simulink model "sampleModel92"  (R2021b)
settings: Solver=VariableStepAuto  StartTime=0.0  StopTime=10.0  RelTol=1e-3
undefined symbols (not defined in the file or in its folder): DiscIntNeverNeededParam, Newton, Raphson
libraries: simulink x6
settings Model: Creator=user  LastModifiedBy=user

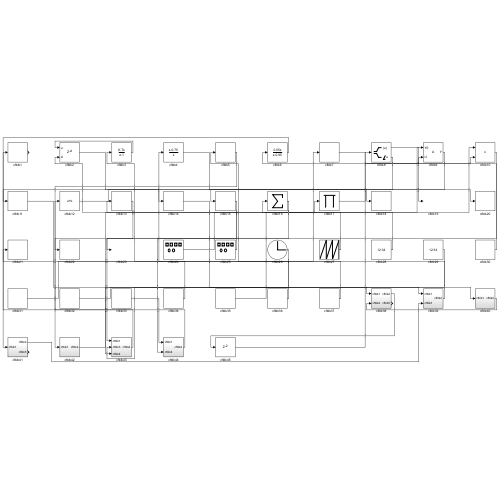
[thumbnail: Simulink's stored preview of the top-level diagram]
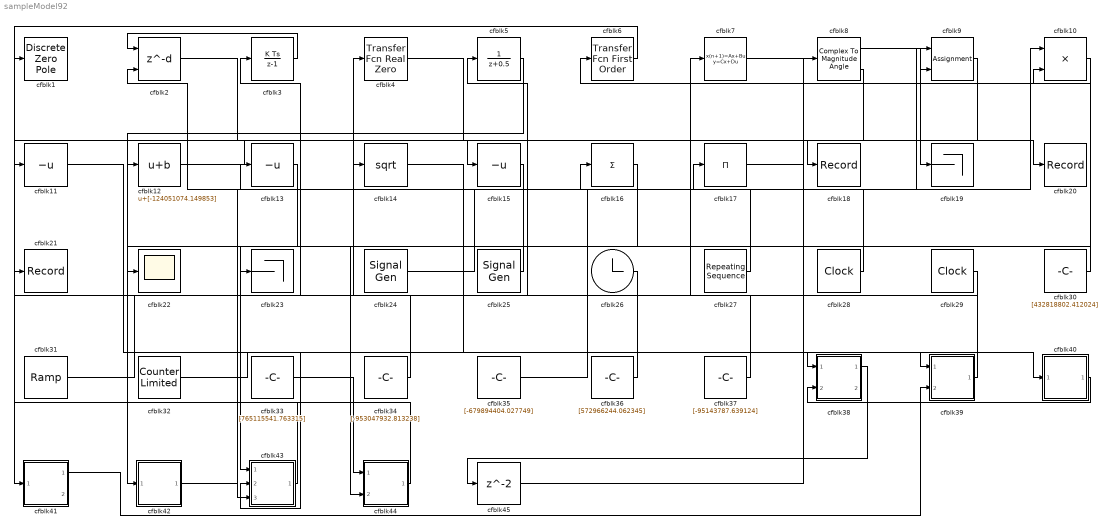
== system sampleModel92 ==
  cfblk1 : DiscreteZeroPole  Poles=[0 0.5]  Gain=1
  cfblk10 : Product
  cfblk11 : UnaryMinus
  cfblk12 : Bias  Bias=[-124051074.149853]
  cfblk13 : UnaryMinus
  cfblk14 : Sqrt  SaturateOnIntegerOverflow=on
  cfblk15 : UnaryMinus
  cfblk16 : Sum  Inputs=+
  cfblk17 : Product  Inputs=*
  cfblk18 : Record  FileSettingsInternal="{\"entries\":[{\"content\":{\"excelSettings\":{\"content\":{},\"type\":\"Streamout.ExcelSettings\"}},\"type\":\"Streamout.FileSettingStorage\",\"uuid\":\"6a51076d-8da9-4467-914a-28448b775d9d\"}],\"packageUris\":[\"http://schema.mathworks.com/mf0/streamout_blocks/R2020a\"],\"version\":\"1.0\"}"  SignalsInternal="{\"entries\":[{\"content\":{\"signals\":[{\"content\":{\"blockPath\":[\"sampleModel92/cfblk18\"],\"channel\":[],\"dimensions\":[1],\"domain\":\"sampleModel92/cfblk18\",\"lineColor\":\"#7e2f8e\",\"plots\":[1],\"port\":1,\"sid\":[\"\"],\"signalID\":3336,\"signalName\":\"cfblk4\"},\"type\":\"RecordBlkView.Signal\",\"uuid\":\"c4f05d71-166b-4c34-8946-7f08c4cc9336\"}]},\"type\":\"RecordBlkView.InputSignals\",\"uuid\":\"7a531b9c-db59-4839-bb56-90dd1c5d6161\"}],\"packageUris\":[\"http://schema.mathworks.com/mf0/streamout_blocks/R2020a\"],\"version\":\"1.0\"}"  VisualizationBindings="{\"sparklinesplugin\":{\"info\":[{\"bindingParametersList\":[],\"subplotID\":1}]}}"
  cfblk19 : Terminator
  cfblk2 : Delay  DelayLengthSource=Input port  SampleTime=1
      settings: InputPortMap=u0,p1
  cfblk20 : Record  FileSettingsInternal="{\"entries\":[{\"content\":{\"excelSettings\":{\"content\":{},\"type\":\"Streamout.ExcelSettings\"}},\"type\":\"Streamout.FileSettingStorage\",\"uuid\":\"9044f618-eb01-48c3-80c5-be2844ab762f\"}],\"packageUris\":[\"http://schema.mathworks.com/mf0/streamout_blocks/R2020a\"],\"version\":\"1.0\"}"  SignalsInternal="{\"entries\":[{\"content\":{\"signals\":[{\"content\":{\"blockPath\":[\"sampleModel92/cfblk20\"],\"channel\":[],\"dimensions\":[1],\"domain\":\"sampleModel92/cfblk20\",\"lineColor\":\"#d95319\",\"plots\":[1],\"port\":1,\"sid\":[\"\"],\"signalID\":3328,\"signalName\":\"cfblk12\"},\"type\":\"RecordBlkView.Signal\",\"uuid\":\"913b886d-d33f-4f21-af18-8c6dc12f15ac\"}]},\"type\":\"RecordBlkView.InputSignals\",\"uuid\":\"b0a329a0-5a63-4f71-bd89-f24f022d2b5e\"}],\"packageUris\":[\"http://schema.mathworks.com/mf0/streamout_blocks/R2020a\"],\"version\":\"1.0\"}"  VisualizationBindings="{\"sparklinesplugin\":{\"info\":[{\"bindingParametersList\":[],\"subplotID\":1}]}}"
  cfblk21 : Record  FileSettingsInternal="{\"entries\":[{\"content\":{\"excelSettings\":{\"content\":{},\"type\":\"Streamout.ExcelSettings\"}},\"type\":\"Streamout.FileSettingStorage\",\"uuid\":\"8f3cd402-b646-49ca-a95d-ee623ab04474\"}],\"packageUris\":[\"http://schema.mathworks.com/mf0/streamout_blocks/R2020a\"],\"version\":\"1.0\"}"  SignalsInternal="{\"entries\":[{\"content\":{\"signals\":[{\"content\":{\"blockPath\":[\"sampleModel92/cfblk21\"],\"channel\":[],\"dimensions\":[1],\"domain\":\"sampleModel92/cfblk21\",\"lineColor\":\"#edb120\",\"plots\":[1],\"port\":1,\"sid\":[\"\"],\"signalID\":3332,\"signalName\":\"cfblk44\"},\"type\":\"RecordBlkView.Signal\",\"uuid\":\"ded4a17a-d02b-4987-8ca6-efb213871c75\"}]},\"type\":\"RecordBlkView.InputSignals\",\"uuid\":\"37dec361-af1f-4bc5-9898-b83d7289465a\"}],\"packageUris\":[\"http://schema.mathworks.com/mf0/streamout_blocks/R2020a\"],\"version\":\"1.0\"}"  VisualizationBindings="{\"sparklinesplugin\":{\"info\":[{\"bindingParametersList\":[],\"subplotID\":1}]}}"
  cfblk22 : Scope
  cfblk23 : Terminator
  cfblk24 : SignalGenerator  WaveForm=square  Amplitude=[-232298427.967946]  Units=rad/sec
  cfblk25 : SignalGenerator  Amplitude=[-137299027.507502]  Units=rad/sec
  cfblk26 : Clock
  cfblk27 : simulink/Sources/Repeating Sequence  rep_seq_t=[0 2]  rep_seq_y=[-945702141.819262, 64967850.415956]
  cfblk28 : DigitalClock
  cfblk29 : DigitalClock
  cfblk3 : DiscreteIntegrator  ICPrevOutput=DiscIntNeverNeededParam  ICPrevScaledInput=DiscIntNeverNeededParam
  cfblk30 : Constant  Value=[432818802.412024]  SampleTime=1
  cfblk31 : simulink/Sources/Ramp  slope=[-2473.565325]  start=[11.966407]  InitialOutput=[854978.820776]
  cfblk32 : simulink/Sources/Counter Limited  uplimit=[365.000000]  tsamp=-1
  cfblk33 : Constant  Value=[765115541.763315]  SampleTime=1
  cfblk34 : Constant  Value=[-953047932.813238]  SampleTime=1
  cfblk35 : Constant  Value=[-679894404.027749]  SampleTime=1
  cfblk36 : Constant  Value=[572966244.062345]  SampleTime=1
  cfblk37 : Constant  Value=[-95143787.639124]  SampleTime=1
  cfblk38 : Subsystem
  cfblk39 : Subsystem
  cfblk4 : simulink/Discrete/Transfer Fcn Real Zero  ZeroZ=0.75  ICPrevInput=0.0  DoSatur=off
      settings: SourceProductBaseCode=SL
  cfblk40 : Subsystem
  cfblk41 : Subsystem
  cfblk42 : Subsystem
  cfblk43 : Subsystem
  cfblk44 : Subsystem
  cfblk45 : Delay  SampleTime=1
  cfblk5 : DiscreteTransferFcn  SampleTime=1
  cfblk6 : simulink/Discrete/Transfer Fcn First Order  PoleZ=0.95  ICPrevOutput=0.0  DoSatur=off
  cfblk7 : DiscreteStateSpace
  cfblk8 : ComplexToMagnitudeAngle
  cfblk9 : Assignment  DiagnosticForDimensions=Warning  IndexOptions=Index vector (dialog)  Indices=1  OutputSizes=1
  wires:
  cfblk12/1 -> cfblk20/1
  cfblk15/1 -> cfblk43/1(cfblk1)
  cfblk30/1 -> cfblk6/1
  cfblk9/1 -> cfblk15/1
  cfblk26/1 -> cfblk43/2(cfblk3)
  cfblk5/1 -> cfblk42/1(cfblk1)
  cfblk24/1 -> cfblk10/1
  cfblk43/1(cfblk2) -> cfblk12/1
  cfblk36/1 -> cfblk5/1
  cfblk29/1 -> cfblk43/3(cfblk4)
  cfblk3/1 -> cfblk2/1
  cfblk8/1 -> cfblk19/1
  cfblk13/1 -> cfblk23/1
  cfblk25/1 -> cfblk13/1
  cfblk35/1 -> cfblk9/1
  cfblk4/1 -> cfblk18/1
  cfblk27/1 -> cfblk2/2
  cfblk6/1 -> cfblk41/1(cfblk1)
  cfblk37/1 -> cfblk1/1
  cfblk10/1 -> cfblk22/1
  cfblk32/1 -> cfblk40/1(cfblk1)
  cfblk28/1 -> cfblk16/1
  cfblk39/1(cfblk2) -> cfblk4/1
  cfblk14/1 -> cfblk39/1(cfblk1)
  cfblk41/1(cfblk2) -> cfblk39/2(cfblk3)
  cfblk34/1 -> cfblk3/1
  cfblk42/1(cfblk2) -> cfblk17/1
  cfblk11/1 -> cfblk38/1(cfblk1)
  cfblk40/1(cfblk2) -> cfblk38/2(cfblk4)
  cfblk31/1 -> cfblk7/1
  cfblk17/1 -> cfblk10/2
  cfblk2/1 -> cfblk14/1
  cfblk33/1 -> cfblk44/1(cfblk1)
  cfblk44/1(cfblk2) -> cfblk21/1
  cfblk7/1 -> cfblk9/2
  cfblk16/1 -> cfblk44/2(cfblk4)
  cfblk8/2 -> cfblk11/1
  cfblk38/1(cfblk2) -> cfblk45/1
  cfblk45/1 -> cfblk8/1

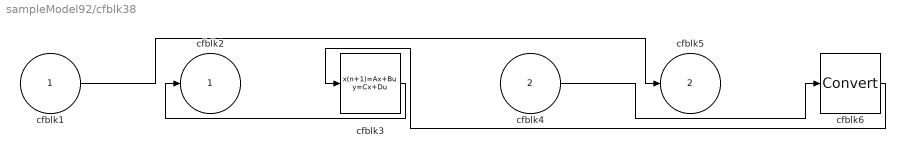
== system sampleModel92/cfblk38 ==
  cfblk1 : Inport
  cfblk4 : Inport  Port=2
  cfblk3 : DiscreteStateSpace
  cfblk6 : DataTypeConversion
  cfblk2 : Outport
  cfblk5 : Outport  Port=2
  wires:
  cfblk3/1 -> cfblk2/1
  cfblk1/1 -> cfblk5/1
  cfblk4/1 -> cfblk6/1
  cfblk6/1 -> cfblk3/1

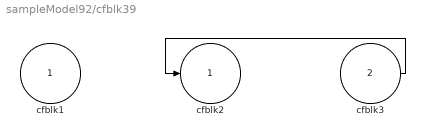
== system sampleModel92/cfblk39 ==
  cfblk1 : Inport
  cfblk3 : Inport  Port=2
  cfblk2 : Outport
  wires:
  cfblk3/1 -> cfblk2/1

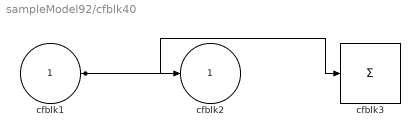
== system sampleModel92/cfblk40 ==
  cfblk1 : Inport
  cfblk3 : Sum  Inputs=+
  cfblk2 : Outport
  wires:
  cfblk1/1 -> cfblk2/1, cfblk3/1

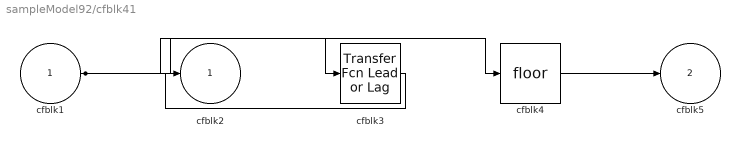
== system sampleModel92/cfblk41 ==
  cfblk1 : Inport
  cfblk3 : simulink/Discrete/Transfer Fcn Lead or Lag  PoleZ=0.95  ZeroZ=0.75  ICPrevOutput=0.0  ICPrevInput=0.0  DoSatur=off
      settings: SourceProductBaseCode=SL
  cfblk4 : Rounding
  cfblk2 : Outport
  cfblk5 : Outport  Port=2
  wires:
  cfblk1/1 -> cfblk4/1, cfblk3/1
  cfblk4/1 -> cfblk5/1
  cfblk3/1 -> cfblk2/1

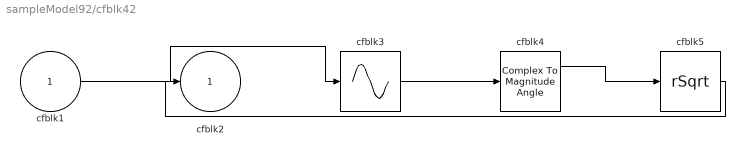
== system sampleModel92/cfblk42 ==
  cfblk1 : Inport
  cfblk3 : Sin  TimeSource=Use external signal  SampleTime=0
  cfblk4 : ComplexToMagnitudeAngle
  cfblk5 : Sqrt  Operator=rSqrt  AlgorithmType=Newton-Raphson  SaturateOnIntegerOverflow=on
  cfblk2 : Outport
  wires:
  cfblk1/1 -> cfblk3/1
  cfblk4/1 -> cfblk5/1
  cfblk3/1 -> cfblk4/1
  cfblk5/1 -> cfblk2/1

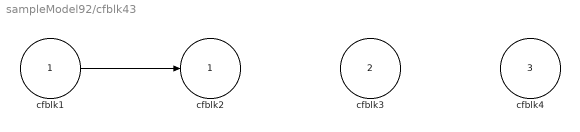
== system sampleModel92/cfblk43 ==
  cfblk1 : Inport
  cfblk3 : Inport  Port=2
  cfblk4 : Inport  Port=3
  cfblk2 : Outport
  wires:
  cfblk1/1 -> cfblk2/1

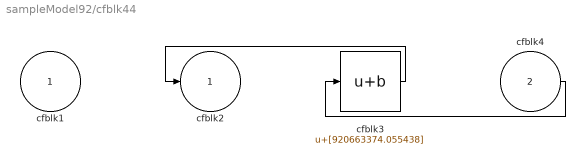
== system sampleModel92/cfblk44 ==
  cfblk1 : Inport
  cfblk4 : Inport  Port=2
  cfblk3 : Bias  Bias=[920663374.055438]
  cfblk2 : Outport
  wires:
  cfblk3/1 -> cfblk2/1
  cfblk4/1 -> cfblk3/1
